simulink model "SF042A_HwAgSnsrls"  (R2013b)
settings: Solver=FixedStepDiscrete  SolverMode=SingleTasking  StartTime=0.0  StopTime=1  FixedStep=0.002  RelTol=1e-3
values from neighbouring files (symbols this model uses):
  ARCHGLBPRM_2MILLISEC_SEC_F32 = DataDict.Constant    [SF042A_HwAgSnsrls_DataDict.m]
  CORRDPINIONAGCON_CNT_U08 = DataDict.Constant    [SF042A_HwAgSnsrls_DataDict.m]
  FCENTROFFSCON_CNT_U08 = DataDict.Constant    [SF042A_HwAgSnsrls_DataDict.m]
  HwAgSnsrlsCorrdPinionAgHwConf = DataDict.Calibration    [SF042A_HwAgSnsrls_DataDict.m]
  HwAgSnsrlsFCentrHwConf = DataDict.Calibration    [SF042A_HwAgSnsrls_DataDict.m]
  HwAgSnsrlsSmotngCoeff = DataDict.Calibration    [SF042A_HwAgSnsrls_DataDict.m]
  HwAgSnsrlsSmotngStepThd = DataDict.Calibration    [SF042A_HwAgSnsrls_DataDict.m]
  HwAgSnsrlsStordPinionConf = DataDict.Calibration    [SF042A_HwAgSnsrls_DataDict.m]
  HwAgSnsrlsStordPinionConfThd = DataDict.Calibration    [SF042A_HwAgSnsrls_DataDict.m]
  HwAgSnsrlsVehDynDifThd = DataDict.Calibration    [SF042A_HwAgSnsrls_DataDict.m]
  HwAgSnsrlsVehDynHwConf = DataDict.Calibration    [SF042A_HwAgSnsrls_DataDict.m]
  HwAgSnsrlsVehDynMotVelThd = DataDict.Calibration    [SF042A_HwAgSnsrls_DataDict.m]
  HwAgSnsrlsVehDynPinionTqThd = DataDict.Calibration    [SF042A_HwAgSnsrls_DataDict.m]
  HwAgSnsrlsVehDynTmr1Thd = DataDict.Calibration    [SF042A_HwAgSnsrls_DataDict.m]
  HwAgSnsrlsVehDynTmr2Thd = DataDict.Calibration    [SF042A_HwAgSnsrls_DataDict.m]
  HwAgSnsrlsVehDynVehSpdThd = DataDict.Calibration    [SF042A_HwAgSnsrls_DataDict.m]
  HwAgSnsrlsVehDynYawRateThd = DataDict.Calibration    [SF042A_HwAgSnsrls_DataDict.m]
  HwAgSnsrlsWhlFrqThd = DataDict.Calibration    [SF042A_HwAgSnsrls_DataDict.m]
  HwAgSnsrlsWhlSpdHwAgCoeff1 = DataDict.Calibration    [SF042A_HwAgSnsrls_DataDict.m]
  HwAgSnsrlsWhlSpdHwAgCoeff2 = DataDict.Calibration    [SF042A_HwAgSnsrls_DataDict.m]
  HwAgSnsrlsWhlSpdHwAgThd = DataDict.Calibration    [SF042A_HwAgSnsrls_DataDict.m]
  HwAgSnsrlsWhlSpdHwConf = DataDict.Calibration    [SF042A_HwAgSnsrls_DataDict.m]
  HwAgSnsrlsWhlSpdRatThd = DataDict.Calibration    [SF042A_HwAgSnsrls_DataDict.m]
  HwAgSnsrlsWhlSpdTmrThd = DataDict.Calibration    [SF042A_HwAgSnsrls_DataDict.m]
  HwAgSnsrlsWhlSpdVehSpdThd = DataDict.Calibration    [SF042A_HwAgSnsrls_DataDict.m]
  LASTPOSNCON_CNT_U08 = DataDict.Constant    [SF042A_HwAgSnsrls_DataDict.m]
  MILLISECTO100MICROSEC_ULS_U32 = DataDict.Constant    [SF042A_HwAgSnsrls_DataDict.m]
  SysGlbPrmSysKineRat = DataDict.ImprtdCal    [SF042A_HwAgSnsrls_DataDict.m]
  SysGlbPrmSysTqRat = DataDict.ImprtdCal    [SF042A_HwAgSnsrls_DataDict.m]
  VEHDYNCON_CNT_U08 = DataDict.Constant    [SF042A_HwAgSnsrls_DataDict.m]
  WHLSPDCON_CNT_U08 = DataDict.Constant    [SF042A_HwAgSnsrls_DataDict.m]
undefined symbols (not defined in the file or in its folder): NtcNr1, SigQlfr1
libraries: NxtrAbslt x11, Fil x8, NxtrLim x4, simulink x3, NxtrNvM x1, FixdToFloat x1
(part 3 of 6)

== system SF042A_HwAgSnsrls/HwAgSnsrls/HwAgSnsrlsPer1/FCentr/If Action Subsystem ==
  RelHwAg : Inport  RequirementInfo={'linktype_rmi_doors' '00012961 (/E-STEER Core/SubSystem Specifications/Application Functions - EA4/SF042A Handwheel Angle Sensorless)' '#SF042A_69' 'true' 'REQ: SF042A_69' '' } %GIDa_4b6aed22_1d87_4b53_9189_d2644312f9f7
  Action Port : ActionPort  ActionType=then
  Constant1 : Constant  RequirementInfo="{'linktype_rmi_doors' '00012961 (/E-STEER Core/SubSystem Specifications/Application Functions - EA4/SF042A Handwheel Angle Sensorless)' '#SF042A_86' 'true' 'REQ:  SF042A_86' '' } %GIDa_2c467a3f_0d7c_4fdb_b837_6c4a5133068f"  Value=HwAgSnsrlsFCentrHwConf
  Constant2 : Constant  RequirementInfo={} %GIDa_675a5498_0baa_424c_b737_c1dad0f0e80d  Value=false  OutDataTypeStr=boolean
      settings: AttributesFormatString=%<OutDataTypeStr>
  CopyRight2 : Subsystem  Description=|  mask(Copyright Information){none=on}
      | Copyright info block.                                               
      |                                                                     
      | Place copyright information at the top of every subsystem in design.
      mask prompts: none "No parameters"
      mask help: Place copyright information at the top of every subsystem in design.
      mask Display:
      | NxtrConf = 'Nexteer Confidential';
      | 
      | sys = bdroot; %handle for the current model ("system")
      | first = get_param(sys,'Created');
      | if(isempty(first))
      |     first = datestr(now,'yyyy');
      | else
      |     first = first(end-3:end);  %year is last four digits
      | end
      | 
      | last = get_param(sys,'LastModifiedDate');
      | if isempty(last)
      |     last = datestr(now,'yyyy');
      | else
      |     last = last(end-3:end);
      | end
      | 
      | if strcmp(first,last)
      |     fprintf('%s -- Copyright %s Nexteer',NxtrConf,first)
      | else
      |     fprintf('%s -- %s%s- %s Nexteer',NxtrConf,char(169),first,last)
      | end
  Data Store Write : DataStoreWrite  RequirementInfo={} %GIDa_7ab1a69a_e36e_4ab1_a11e_792ec32a2170  DataStoreName=FCentrHwAgEna
  Data Store Write1 : DataStoreWrite  RequirementInfo={'linktype_rmi_doors' '00012961 (/E-STEER Core/SubSystem Specifications/Application Functions - EA4/SF042A Handwheel Angle Sensorless)' '#SF042A_69' 'true' 'REQ: SF042A_69' '' } %GIDa_34d06627_b66b_4ac4_8bdd_291c574c45f0  DataStoreName=FCentrHwAgOffs
  Data Store Write2 : DataStoreWrite  RequirementInfo="{'linktype_rmi_doors' '00012961 (/E-STEER Core/SubSystem Specifications/Application Functions - EA4/SF042A Handwheel Angle Sensorless)' '#SF042A_86' 'true' 'REQ:  SF042A_86' '' } %GIDa_6b896a4e_80c9_41a2_80ba_aa37785d56f0"  DataStoreName=FCentrHwConf
  wires:
  Constant1/1 -> Data Store Write2/1
  Constant2/1 -> Data Store Write/1
  RelHwAg/1 -> Data Store Write1/1

== system SF042A_HwAgSnsrls/HwAgSnsrls/HwAgSnsrlsPer1/RelHwAgCalcn/CopyRight2 ==

== system SF042A_HwAgSnsrls/HwAgSnsrls/HwAgSnsrlsPer1/RelHwAgCalcn/Set to 0 ==
  Action Port : ActionPort  ActionType=else
  Constant1 : Constant  RequirementInfo={} %GIDa_94a063b7_dc94_4966_ace2_3847eccd81e4  Value=0  OutDataTypeStr=single
      settings: AttributesFormatString=%<OutDataTypeStr>
  CopyRight2 : Subsystem  Description=|  mask(Copyright Information){none=on}
      | Copyright info block.                                               
      |                                                                     
      | Place copyright information at the top of every subsystem in design.
      mask prompts: none "No parameters"
      mask help: Place copyright information at the top of every subsystem in design.
      mask Display:
      | NxtrConf = 'Nexteer Confidential';
      | 
      | sys = bdroot; %handle for the current model ("system")
      | first = get_param(sys,'Created');
      | if(isempty(first))
      |     first = datestr(now,'yyyy');
      | else
      |     first = first(end-3:end);  %year is last four digits
      | end
      | 
      | last = get_param(sys,'LastModifiedDate');
      | if isempty(last)
      |     last = datestr(now,'yyyy');
      | else
      |     last = last(end-3:end);
      | end
      | 
      | if strcmp(first,last)
      |     fprintf('%s -- Copyright %s Nexteer',NxtrConf,first)
      | else
      |     fprintf('%s -- %s%s- %s Nexteer',NxtrConf,char(169),first,last)
      | end
  Out1 : Outport
  wires:
  Constant1/1 -> Out1/1

== system SF042A_HwAgSnsrls/HwAgSnsrls/HwAgSnsrlsPer1/RelHwAgCalcn/UseMotAg ==
  MotAgCumvAlgndCrf : Inport
  Action Port : ActionPort  ActionType=then
  CopyRight2 : Subsystem  Description=|  mask(Copyright Information){none=on}
      | Copyright info block.                                               
      |                                                                     
      | Place copyright information at the top of every subsystem in design.
      mask prompts: none "No parameters"
      mask help: Place copyright information at the top of every subsystem in design.
      mask Display:
      | NxtrConf = 'Nexteer Confidential';
      | 
      | sys = bdroot; %handle for the current model ("system")
      | first = get_param(sys,'Created');
      | if(isempty(first))
      |     first = datestr(now,'yyyy');
      | else
      |     first = first(end-3:end);  %year is last four digits
      | end
      | 
      | last = get_param(sys,'LastModifiedDate');
      | if isempty(last)
      |     last = datestr(now,'yyyy');
      | else
      |     last = last(end-3:end);
      | end
      | 
      | if strcmp(first,last)
      |     fprintf('%s -- Copyright %s Nexteer',NxtrConf,first)
      | else
      |     fprintf('%s -- %s%s- %s Nexteer',NxtrConf,char(169),first,last)
      | end
  Data Store Read2 : DataStoreRead  DataStoreName=MotAgOffsEna
  GetMotAgOffs : Subsystem  TreatAsAtomicUnit=on
  If : If  IfExpression=u1  ShowElse=off
  Out1 : Outport
  wires:
  MotAgCumvAlgndCrf/1 -> GetMotAgOffs/1(In1), Out1/1
  Data Store Read2/1 -> If/1
  If/1 -> GetMotAgOffs/Action

== system SF042A_HwAgSnsrls/HwAgSnsrls/HwAgSnsrlsPer1/Smoothing/CopyRight2 ==

== system SF042A_HwAgSnsrls/HwAgSnsrls/HwAgSnsrlsPer1/Smoothing/If Action Subsystem ==
  LrndHwAgDif : Inport
  Action Port : ActionPort  ActionType=then
  Add1 : Sum
  Constant1 : Constant  Value=true  OutDataTypeStr=boolean
  Constant3 : Constant  Value=HwAgSnsrlsSmotngCoeff
  CopyRight2 : Subsystem  Description=|  mask(Copyright Information){none=on}
      | Copyright info block.                                               
      |                                                                     
      | Place copyright information at the top of every subsystem in design.
      mask prompts: none "No parameters"
      mask help: Place copyright information at the top of every subsystem in design.
      mask Display:
      | NxtrConf = 'Nexteer Confidential';
      | 
      | sys = bdroot; %handle for the current model ("system")
      | first = get_param(sys,'Created');
      | if(isempty(first))
      |     first = datestr(now,'yyyy');
      | else
      |     first = first(end-3:end);  %year is last four digits
      | end
      | 
      | last = get_param(sys,'LastModifiedDate');
      | if isempty(last)
      |     last = datestr(now,'yyyy');
      | else
      |     last = last(end-3:end);
      | end
      | 
      | if strcmp(first,last)
      |     fprintf('%s -- Copyright %s Nexteer',NxtrConf,first)
      | else
      |     fprintf('%s -- %s%s- %s Nexteer',NxtrConf,char(169),first,last)
      | end
  Data Store Read2 : DataStoreRead  DataStoreName=PrevSmotngHwAg
  Data Store Write1 : DataStoreWrite  DataStoreName=PrevSmotngSt
  Product2 : Product
  Outp : Outport
  wires:
  Add1/1 -> Outp/1
  Product2/1 -> Add1/1
  Data Store Read2/1 -> Add1/2
  Constant3/1 -> Product2/2
  Constant1/1 -> Data Store Write1/1
  LrndHwAgDif/1 -> Product2/1

== system SF042A_HwAgSnsrls/HwAgSnsrls/HwAgSnsrlsPer1/Smoothing/If Action Subsystem1 ==
  LrndHwAg : Inport
  Action Port : ActionPort  ActionType=else
  Constant1 : Constant  Value=false  OutDataTypeStr=boolean
  CopyRight2 : Subsystem  Description=|  mask(Copyright Information){none=on}
      | Copyright info block.                                               
      |                                                                     
      | Place copyright information at the top of every subsystem in design.
      mask prompts: none "No parameters"
      mask help: Place copyright information at the top of every subsystem in design.
      mask Display:
      | NxtrConf = 'Nexteer Confidential';
      | 
      | sys = bdroot; %handle for the current model ("system")
      | first = get_param(sys,'Created');
      | if(isempty(first))
      |     first = datestr(now,'yyyy');
      | else
      |     first = first(end-3:end);  %year is last four digits
      | end
      | 
      | last = get_param(sys,'LastModifiedDate');
      | if isempty(last)
      |     last = datestr(now,'yyyy');
      | else
      |     last = last(end-3:end);
      | end
      | 
      | if strcmp(first,last)
      |     fprintf('%s -- Copyright %s Nexteer',NxtrConf,first)
      | else
      |     fprintf('%s -- %s%s- %s Nexteer',NxtrConf,char(169),first,last)
      | end
  Data Store Write1 : DataStoreWrite  DataStoreName=PrevSmotngSt
  Outp : Outport
  wires:
  LrndHwAg/1 -> Outp/1
  Constant1/1 -> Data Store Write1/1

== system SF042A_HwAgSnsrls/HwAgSnsrls/HwAgSnsrlsPer1/VehDynAutoCentr/CopyRight2 ==

== system SF042A_HwAgSnsrls/HwAgSnsrls/HwAgSnsrlsPer1/VehDynAutoCentr/LpFilOne ==
  FilOneEna : Inport
  RelHwAg : Inport  Port=2
  CopyRight2 : Subsystem  Description=|  mask(Copyright Information){none=on}
      | Copyright info block.                                               
      |                                                                     
      | Place copyright information at the top of every subsystem in design.
      mask prompts: none "No parameters"
      mask help: Place copyright information at the top of every subsystem in design.
      mask Display:
      | NxtrConf = 'Nexteer Confidential';
      | 
      | sys = bdroot; %handle for the current model ("system")
      | first = get_param(sys,'Created');
      | if(isempty(first))
      |     first = datestr(now,'yyyy');
      | else
      |     first = first(end-3:end);  %year is last four digits
      | end
      | 
      | last = get_param(sys,'LastModifiedDate');
      | if isempty(last)
      |     last = datestr(now,'yyyy');
      | else
      |     last = last(end-3:end);
      | end
      | 
      | if strcmp(first,last)
      |     fprintf('%s -- Copyright %s Nexteer',NxtrConf,first)
      | else
      |     fprintf('%s -- %s%s- %s Nexteer',NxtrConf,char(169),first,last)
      | end
  Data Store Write : DataStoreWrite  DataStoreName=PrevFildRelHwAg1
  If : If  RequirementInfo={'linktype_rmi_doors' '00012961 (/E-STEER Core/SubSystem Specifications/Application Functions - EA4/SF042A Handwheel Angle Sensorless)' '#SF042A_74' 'true' 'REQ: SF042A_74' '' } %GIDa_50dbe270_ec98_43d4_9cbb_cd5ecb0c86de  IfExpression=u1
  If Action Subsystem1 : Subsystem  RequirementInfo={'linktype_rmi_doors' '00012961 (/E-STEER Core/SubSystem Specifications/Application Functions - EA4/SF042A Handwheel Angle Sensorless)' '#SF042A_74' 'true' 'REQ: SF042A_74' '' } %GIDa_d396f57d_b9c8_4c45_ae6c_b596f7fbf48d  TreatAsAtomicUnit=on
  If Action Subsystem2 : Subsystem  RequirementInfo={'linktype_rmi_doors' '00012961 (/E-STEER Core/SubSystem Specifications/Application Functions - EA4/SF042A Handwheel Angle Sensorless)' '#SF042A_74' 'true' 'REQ: SF042A_74' '' } %GIDa_038cab70_eae8_4b9a_8597_cbcafc370d1a  TreatAsAtomicUnit=on
  Merge : Merge  RequirementInfo={'linktype_rmi_doors' '00012961 (/E-STEER Core/SubSystem Specifications/Application Functions - EA4/SF042A Handwheel Angle Sensorless)' '#SF042A_74' 'true' 'REQ: SF042A_74' '' } %GIDa_64de599a_2316_4355_972d_e88e49288b80
  FildRelHwAg1 : Outport
  wires:
  Merge/1 -> FildRelHwAg1/1, Data Store Write/1
  FilOneEna/1 -> If/1
  RelHwAg/1 -> If Action Subsystem2/1(RelHwAg)
  If Action Subsystem2/1(FildRelHwAg1) -> Merge/1
  If Action Subsystem1/1(FildRelHwAg1) -> Merge/2
  If/2 -> If Action Subsystem1/Action
  If/1 -> If Action Subsystem2/Action

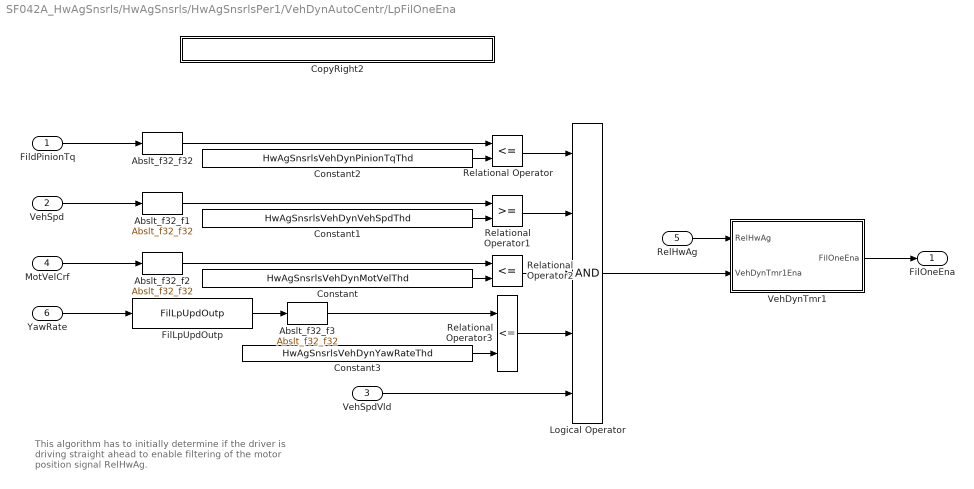
== system SF042A_HwAgSnsrls/HwAgSnsrls/HwAgSnsrlsPer1/VehDynAutoCentr/LpFilOneEna ==
  note: This algorithm has to initially determine if the driver is
      | driving straight ahead to enable filtering of the motor
      | position signal RelHwAg.
  FildPinionTq : Inport
  VehSpd : Inport  Port=2
  VehSpdVld : Inport  Port=3
  MotVelCrf : Inport  Port=4
  RelHwAg : Inport  Port=5
  YawRate : Inport  Port=6
  Abslt_f32_f1 : NxtrAbslt/Abslt_f32_f32  RequirementInfo={'linktype_rmi_doors' '00012961 (/E-STEER Core/SubSystem Specifications/Application Functions - EA4/SF042A Handwheel Angle Sensorless)' '#SF042A_73' 'true' 'REQ: SF042A_73' '' } %GIDa_47b4a5eb_74c9_48e6_977d_5f1b477ad6dd  SFunctionSpec=single y1 = Abslt_f32_f32(single u1)
      settings: AttributesFormatString=%<Name>
  Abslt_f32_f2 : NxtrAbslt/Abslt_f32_f32  RequirementInfo={'linktype_rmi_doors' '00012961 (/E-STEER Core/SubSystem Specifications/Application Functions - EA4/SF042A Handwheel Angle Sensorless)' '#SF042A_73' 'true' 'REQ: SF042A_73' '' } %GIDa_ea5515ef_69f8_4e78_8562_cc1ad73cd76b  SFunctionSpec=single y1 = Abslt_f32_f32(single u1)
      settings: AttributesFormatString=%<Name>
  Abslt_f32_f3 : NxtrAbslt/Abslt_f32_f32  RequirementInfo={'linktype_rmi_doors' '00012961 (/E-STEER Core/SubSystem Specifications/Application Functions - EA4/SF042A Handwheel Angle Sensorless)' '#SF042A_73' 'true' 'REQ: SF042A_73' '' } %GIDa_70050457_0f45_4f04_b196_a55d8517b918  SFunctionSpec=single y1 = Abslt_f32_f32(single u1)
      settings: AttributesFormatString=%<Name>
  Abslt_f32_f32 : NxtrAbslt/Abslt_f32_f32  RequirementInfo={'linktype_rmi_doors' '00012961 (/E-STEER Core/SubSystem Specifications/Application Functions - EA4/SF042A Handwheel Angle Sensorless)' '#SF042A_73' 'true' 'REQ: SF042A_73' '' } %GIDa_f624d835_a012_455e_a6e7_bf5bbda701df  SFunctionSpec=single y1 = Abslt_f32_f32(single u1)
      settings: AttributesFormatString=%<Name>
  Constant : Constant  RequirementInfo={'linktype_rmi_doors' '00012961 (/E-STEER Core/SubSystem Specifications/Application Functions - EA4/SF042A Handwheel Angle Sensorless)' '#SF042A_73' 'true' 'REQ: SF042A_73' '' } %GIDa_33de20e7_381d_4057_a25e_061ade792d0e  Value=HwAgSnsrlsVehDynMotVelThd
  Constant1 : Constant  RequirementInfo={'linktype_rmi_doors' '00012961 (/E-STEER Core/SubSystem Specifications/Application Functions - EA4/SF042A Handwheel Angle Sensorless)' '#SF042A_73' 'true' 'REQ: SF042A_73' '' } %GIDa_7455e53e_a0fa_4ad3_9554_8a19bfe16525  Value=HwAgSnsrlsVehDynVehSpdThd
  Constant2 : Constant  RequirementInfo={'linktype_rmi_doors' '00012961 (/E-STEER Core/SubSystem Specifications/Application Functions - EA4/SF042A Handwheel Angle Sensorless)' '#SF042A_73' 'true' 'REQ: SF042A_73' '' } %GIDa_60d6fec9_a19e_4266_9b3b_fb17078d585a  Value=HwAgSnsrlsVehDynPinionTqThd
  Constant3 : Constant  RequirementInfo={'linktype_rmi_doors' '00012961 (/E-STEER Core/SubSystem Specifications/Application Functions - EA4/SF042A Handwheel Angle Sensorless)' '#SF042A_73' 'true' 'REQ: SF042A_73' '' } %GIDa_08b4b183_3ae9_45ec_b5d2_fc4ee1e02481  Value=HwAgSnsrlsVehDynYawRateThd
  CopyRight2 : Subsystem  Description=|  mask(Copyright Information){none=on}
      | Copyright info block.                                               
      |                                                                     
      | Place copyright information at the top of every subsystem in design.
      mask prompts: none "No parameters"
      mask help: Place copyright information at the top of every subsystem in design.
      mask Display:
      | NxtrConf = 'Nexteer Confidential';
      | 
      | sys = bdroot; %handle for the current model ("system")
      | first = get_param(sys,'Created');
      | if(isempty(first))
      |     first = datestr(now,'yyyy');
      | else
      |     first = first(end-3:end);  %year is last four digits
      | end
      | 
      | last = get_param(sys,'LastModifiedDate');
      | if isempty(last)
      |     last = datestr(now,'yyyy');
      | else
      |     last = last(end-3:end);
      | end
      | 
      | if strcmp(first,last)
      |     fprintf('%s -- Copyright %s Nexteer',NxtrConf,first)
      | else
      |     fprintf('%s -- %s%s- %s Nexteer',NxtrConf,char(169),first,last)
      | end
  FilLpUpdOutp : Fil/FilLpUpdOutp  RequirementInfo={'linktype_rmi_doors' '00012961 (/E-STEER Core/SubSystem Specifications/Application Functions - EA4/SF042A Handwheel Angle Sensorless)' '#SF042A_73' 'true' 'REQ: SF042A_73' '' } %GIDa_2485b240_b275_4f39_b29a_c03896a8b7bb  StVar=YawRateFil
      settings: AttributesFormatString=StVar: %<StVar>
  Logical Operator : Logic  RequirementInfo={'linktype_rmi_doors' '00012961 (/E-STEER Core/SubSystem Specifications/Application Functions - EA4/SF042A Handwheel Angle Sensorless)' '#SF042A_73' 'true' 'REQ: SF042A_73' '' } %GIDa_490bb6e2_0097_4fb5_8883_f3aba4d42fa5  Inputs=5  AllPortsSameDT=off  OutDataTypeStr=boolean
  Relational Operator : RelationalOperator  RequirementInfo={'linktype_rmi_doors' '00012961 (/E-STEER Core/SubSystem Specifications/Application Functions - EA4/SF042A Handwheel Angle Sensorless)' '#SF042A_73' 'true' 'REQ: SF042A_73' '' } %GIDa_f6893bfc_cdd3_4f77_af64_1f833848b7e5  Operator=<=  OutDataTypeStr=boolean
  Relational Operator1 : RelationalOperator  RequirementInfo={'linktype_rmi_doors' '00012961 (/E-STEER Core/SubSystem Specifications/Application Functions - EA4/SF042A Handwheel Angle Sensorless)' '#SF042A_73' 'true' 'REQ: SF042A_73' '' } %GIDa_8a3715e6_0a30_4e30_a0ce_0eaccb932bbf  OutDataTypeStr=boolean
  Relational Operator2 : RelationalOperator  RequirementInfo={'linktype_rmi_doors' '00012961 (/E-STEER Core/SubSystem Specifications/Application Functions - EA4/SF042A Handwheel Angle Sensorless)' '#SF042A_73' 'true' 'REQ: SF042A_73' '' } %GIDa_3da8d1a4_697d_4093_b262_91d6ea858a11  Operator=<=  OutDataTypeStr=boolean
  Relational Operator3 : RelationalOperator  RequirementInfo={'linktype_rmi_doors' '00012961 (/E-STEER Core/SubSystem Specifications/Application Functions - EA4/SF042A Handwheel Angle Sensorless)' '#SF042A_73' 'true' 'REQ: SF042A_73' '' } %GIDa_40a0aebf_3696_464f_8498_1d8daec05661  Operator=<=  OutDataTypeStr=boolean
  VehDynTmr1 : Subsystem  RequirementInfo={'linktype_rmi_doors' '00012961 (/E-STEER Core/SubSystem Specifications/Application Functions - EA4/SF042A Handwheel Angle Sensorless)' '#SF042A_73' 'true' 'REQ: SF042A_73' '' } %GIDa_9b420d72_230e_42ee_a755_3d84b38ed0e9
  FilOneEna : Outport
  wires:
  Abslt_f32_f3/1 -> Relational Operator3/1
  VehSpdVld/1 -> Logical Operator/5
  Constant3/1 -> Relational Operator3/2
  FilLpUpdOutp/1 -> Abslt_f32_f3/1
  YawRate/1 -> FilLpUpdOutp/1
  Logical Operator/1 -> VehDynTmr1/2(VehDynTmr1Ena)
  VehDynTmr1/1(FilOneEna) -> FilOneEna/1
  RelHwAg/1 -> VehDynTmr1/1(RelHwAg)
  Relational Operator2/1 -> Logical Operator/3
  Relational Operator1/1 -> Logical Operator/2
  Relational Operator/1 -> Logical Operator/1
  Relational Operator3/1 -> Logical Operator/4
  Abslt_f32_f2/1 -> Relational Operator2/1
  Constant/1 -> Relational Operator2/2
  Abslt_f32_f1/1 -> Relational Operator1/1
  Constant1/1 -> Relational Operator1/2
  VehSpd/1 -> Abslt_f32_f1/1
  Abslt_f32_f32/1 -> Relational Operator/1
  Constant2/1 -> Relational Operator/2
  MotVelCrf/1 -> Abslt_f32_f2/1
  FildPinionTq/1 -> Abslt_f32_f32/1

== system SF042A_HwAgSnsrls/HwAgSnsrls/HwAgSnsrlsPer1/VehDynAutoCentr/LpFilTwo ==
  note: The output, VehDynHwAg is removed.
      | The display, dHwAgSnsrlsVehDynHwAg is removed.
      | The PIM, PrevFildRelHwAg2 is removed.
  FilTwoEna : Inport
  RelHwAg : Inport  Port=2
  CopyRight2 : Subsystem  Description=|  mask(Copyright Information){none=on}
      | Copyright info block.                                               
      |                                                                     
      | Place copyright information at the top of every subsystem in design.
      mask prompts: none "No parameters"
      mask help: Place copyright information at the top of every subsystem in design.
      mask Display:
      | NxtrConf = 'Nexteer Confidential';
      | 
      | sys = bdroot; %handle for the current model ("system")
      | first = get_param(sys,'Created');
      | if(isempty(first))
      |     first = datestr(now,'yyyy');
      | else
      |     first = first(end-3:end);  %year is last four digits
      | end
      | 
      | last = get_param(sys,'LastModifiedDate');
      | if isempty(last)
      |     last = datestr(now,'yyyy');
      | else
      |     last = last(end-3:end);
      | end
      | 
      | if strcmp(first,last)
      |     fprintf('%s -- Copyright %s Nexteer',NxtrConf,first)
      | else
      |     fprintf('%s -- %s%s- %s Nexteer',NxtrConf,char(169),first,last)
      | end
  Data Store Write1 : DataStoreWrite  DataStoreName=dHwAgSnsrlsVehDynHwConf
  If Action Subsystem3 : Subsystem  RequirementInfo={'linktype_rmi_doors' '00012961 (/E-STEER Core/SubSystem Specifications/Application Functions - EA4/SF042A Handwheel Angle Sensorless)' '#SF042A_76' 'true' 'REQ: SF042A_76' '' } %GIDa_7c18b11c_08c4_4ee8_9dc5_2a8c731949f7  TreatAsAtomicUnit=on
  If Action Subsystem4 : Subsystem  RequirementInfo={'linktype_rmi_doors' '00012961 (/E-STEER Core/SubSystem Specifications/Application Functions - EA4/SF042A Handwheel Angle Sensorless)' '#SF042A_77' 'true' 'REQ: SF042A_77' '' } %GIDa_7dd1b9c8_568d_422e_9620_51905b8cb554  TreatAsAtomicUnit=on
  If1 : If  RequirementInfo={'linktype_rmi_doors' '00012961 (/E-STEER Core/SubSystem Specifications/Application Functions - EA4/SF042A Handwheel Angle Sensorless)' '#SF042A_76' 'true' 'REQ: SF042A_76' '' ; 'linktype_rmi_doors' '00012961 (/E-STEER Core/SubSystem Specifications/Application Functions - EA4/SF042A Handwheel Angle Sensorless)' '#SF042A_77' 'true' 'REQ: SF042A_77' '' } %GIDa_16361238_c0a5_470c_9b94_2028cab79145  IfExpression=u1
  Merge2 : Merge  RequirementInfo={'linktype_rmi_doors' '00012961 (/E-STEER Core/SubSystem Specifications/Application Functions - EA4/SF042A Handwheel Angle Sensorless)' '#SF042A_76' 'true' 'REQ: SF042A_76' '' ; 'linktype_rmi_doors' '00012961 (/E-STEER Core/SubSystem Specifications/Application Functions - EA4/SF042A Handwheel Angle Sensorless)' '#SF042A_77' 'true' 'REQ: SF042A_77' '' } %GIDa_e93193e5_4d94_47be_88ff_d96e66fc9642
  VehDynHwConf : Outport
  wires:
  Merge2/1 -> VehDynHwConf/1, Data Store Write1/1
  If Action Subsystem4/1(VehDynHwConf) -> Merge2/1
  If Action Subsystem3/1(VehDynHwConf) -> Merge2/2
  FilTwoEna/1 -> If1/1
  RelHwAg/1 -> If Action Subsystem4/1(RelHwAg)
  If1/1 -> If Action Subsystem4/Action
  If1/2 -> If Action Subsystem3/Action

== system SF042A_HwAgSnsrls/HwAgSnsrls/HwAgSnsrlsPer1/VehDynAutoCentr/LpFilTwoEna ==
  FildRelHwAg1 : Inport
  RelHwAg : Inport  Port=2
  FilOneEna : Inport  Port=3
  Abslt_f32_f3 : NxtrAbslt/Abslt_f32_f32  RequirementInfo={'linktype_rmi_doors' '00012961 (/E-STEER Core/SubSystem Specifications/Application Functions - EA4/SF042A Handwheel Angle Sensorless)' '#SF042A_75' 'true' 'REQ: SF042A_75' '' } %GIDa_6aeccc63_8826_4a9a_b358_b34695279e3a  SFunctionSpec=single y1 = Abslt_f32_f32(single u1)
      settings: AttributesFormatString=%<Name>
  Add : Sum  RequirementInfo={'linktype_rmi_doors' '00012961 (/E-STEER Core/SubSystem Specifications/Application Functions - EA4/SF042A Handwheel Angle Sensorless)' '#SF042A_75' 'true' 'REQ: SF042A_75' '' } %GIDa_bed5965e_f792_4fe9_be9c_a249f6adb978  Inputs=-+
  Constant5 : Constant  RequirementInfo={'linktype_rmi_doors' '00012961 (/E-STEER Core/SubSystem Specifications/Application Functions - EA4/SF042A Handwheel Angle Sensorless)' '#SF042A_75' 'true' 'REQ: SF042A_75' '' } %GIDa_4312dcf7_970c_416a_83c8_6d334342d5f4  Value=HwAgSnsrlsVehDynDifThd
  CopyRight2 : Subsystem  Description=|  mask(Copyright Information){none=on}
      | Copyright info block.                                               
      |                                                                     
      | Place copyright information at the top of every subsystem in design.
      mask prompts: none "No parameters"
      mask help: Place copyright information at the top of every subsystem in design.
      mask Display:
      | NxtrConf = 'Nexteer Confidential';
      | 
      | sys = bdroot; %handle for the current model ("system")
      | first = get_param(sys,'Created');
      | if(isempty(first))
      |     first = datestr(now,'yyyy');
      | else
      |     first = first(end-3:end);  %year is last four digits
      | end
      | 
      | last = get_param(sys,'LastModifiedDate');
      | if isempty(last)
      |     last = datestr(now,'yyyy');
      | else
      |     last = last(end-3:end);
      | end
      | 
      | if strcmp(first,last)
      |     fprintf('%s -- Copyright %s Nexteer',NxtrConf,first)
      | else
      |     fprintf('%s -- %s%s- %s Nexteer',NxtrConf,char(169),first,last)
      | end
  Logical Operator1 : Logic  RequirementInfo={'linktype_rmi_doors' '00012961 (/E-STEER Core/SubSystem Specifications/Application Functions - EA4/SF042A Handwheel Angle Sensorless)' '#SF042A_75' 'true' 'REQ: SF042A_75' '' } %GIDa_69a84b1a_4e75_466e_ae3a_2b9fc6914824  AllPortsSameDT=off  OutDataTypeStr=boolean
  Relational Operator3 : RelationalOperator  RequirementInfo={'linktype_rmi_doors' '00012961 (/E-STEER Core/SubSystem Specifications/Application Functions - EA4/SF042A Handwheel Angle Sensorless)' '#SF042A_75' 'true' 'REQ: SF042A_75' '' } %GIDa_439f62f5_372d_47fa_800c_5b377eb6c5df  Operator=<=  OutDataTypeStr=boolean
  VehDynTmr2 : Subsystem  RequirementInfo={'linktype_rmi_doors' '00012961 (/E-STEER Core/SubSystem Specifications/Application Functions - EA4/SF042A Handwheel Angle Sensorless)' '#SF042A_75' 'true' 'REQ: SF042A_75' '' } %GIDa_bc352537_dcd2_4910_87c3_9f7bc64451ab
  FilTwoEna : Outport
  wires:
  FildRelHwAg1/1 -> Add/1, [FildRelHwAg1]
  VehDynTmr2/1(FilTwoEna) -> FilTwoEna/1
  [FildRelHwAg1] -> VehDynTmr2/1(FildRelHwAg1)
  Logical Operator1/1 -> VehDynTmr2/2(VehDynTmr2Ena)
  FilOneEna/1 -> Logical Operator1/2
  Relational Operator3/1 -> Logical Operator1/1
  Constant5/1 -> Relational Operator3/2
  Abslt_f32_f3/1 -> Relational Operator3/1
  Add/1 -> Abslt_f32_f3/1
  RelHwAg/1 -> Add/2

== system SF042A_HwAgSnsrls/HwAgSnsrls/HwAgSnsrlsPer1/VehDynAutoCentr/PinionTqCalc ==
  HwTq : Inport
  MotTqCmdCrf : Inport  Port=2
  Add : Sum  RequirementInfo={'linktype_rmi_doors' '00012961 (/E-STEER Core/SubSystem Specifications/Application Functions - EA4/SF042A Handwheel Angle Sensorless)' '#SF042A_67' 'true' 'REQ: SF042A_67' '' } %GIDa_29639fb6_7c22_449f_aaa9_e717a68ba06e
  Constant : Constant  RequirementInfo={'linktype_rmi_doors' '00012961 (/E-STEER Core/SubSystem Specifications/Application Functions - EA4/SF042A Handwheel Angle Sensorless)' '#SF042A_67' 'true' 'REQ: SF042A_67' '' } %GIDa_ce2a4e4e_2b87_4ac6_9ab1_d2b13d4c852e  Value=SysGlbPrmSysTqRat
  CopyRight2 : Subsystem  Description=|  mask(Copyright Information){none=on}
      | Copyright info block.                                               
      |                                                                     
      | Place copyright information at the top of every subsystem in design.
      mask prompts: none "No parameters"
      mask help: Place copyright information at the top of every subsystem in design.
      mask Display:
      | NxtrConf = 'Nexteer Confidential';
      | 
      | sys = bdroot; %handle for the current model ("system")
      | first = get_param(sys,'Created');
      | if(isempty(first))
      |     first = datestr(now,'yyyy');
      | else
      |     first = first(end-3:end);  %year is last four digits
      | end
      | 
      | last = get_param(sys,'LastModifiedDate');
      | if isempty(last)
      |     last = datestr(now,'yyyy');
      | else
      |     last = last(end-3:end);
      | end
      | 
      | if strcmp(first,last)
      |     fprintf('%s -- Copyright %s Nexteer',NxtrConf,first)
      | else
      |     fprintf('%s -- %s%s- %s Nexteer',NxtrConf,char(169),first,last)
      | end
  FilLpUpdOutp : Fil/FilLpUpdOutp  RequirementInfo={'linktype_rmi_doors' '00012961 (/E-STEER Core/SubSystem Specifications/Application Functions - EA4/SF042A Handwheel Angle Sensorless)' '#SF042A_67' 'true' 'REQ: SF042A_67' '' } %GIDa_71b12ad7_8a05_45a2_a00d_d65e9feee573  StVar=PinionTqFil
      settings: AttributesFormatString=StVar: %<StVar>
  Product : Product  RequirementInfo={'linktype_rmi_doors' '00012961 (/E-STEER Core/SubSystem Specifications/Application Functions - EA4/SF042A Handwheel Angle Sensorless)' '#SF042A_67' 'true' 'REQ: SF042A_67' '' } %GIDa_12316cbc_e5f8_4b38_99f2_690332d89a1e
  FildPinionTq : Outport
  wires:
  Constant/1 -> Product/2
  FilLpUpdOutp/1 -> FildPinionTq/1
  Add/1 -> FilLpUpdOutp/1
  HwTq/1 -> Add/1
  Product/1 -> Add/2
  MotTqCmdCrf/1 -> Product/1

== system SF042A_HwAgSnsrls/HwAgSnsrls/HwAgSnsrlsPer1/WhlSpdAutoCentr/CopyRight2 ==

== system SF042A_HwAgSnsrls/HwAgSnsrls/HwAgSnsrlsPer1/WhlSpdAutoCentr/WhlFrqNotVld ==
  note: The output, WhlSpdHwAg, is removed.
  Action Port : ActionPort  ActionType=else
  Constant1 : Constant  Value=0  OutDataTypeStr=single
      settings: AttributesFormatString=%<OutDataTypeStr>
  CopyRight2 : Subsystem  Description=|  mask(Copyright Information){none=on}
      | Copyright info block.                                               
      |                                                                     
      | Place copyright information at the top of every subsystem in design.
      mask prompts: none "No parameters"
      mask help: Place copyright information at the top of every subsystem in design.
      mask Display:
      | NxtrConf = 'Nexteer Confidential';
      | 
      | sys = bdroot; %handle for the current model ("system")
      | first = get_param(sys,'Created');
      | if(isempty(first))
      |     first = datestr(now,'yyyy');
      | else
      |     first = first(end-3:end);  %year is last four digits
      | end
      | 
      | last = get_param(sys,'LastModifiedDate');
      | if isempty(last)
      |     last = datestr(now,'yyyy');
      | else
      |     last = last(end-3:end);
      | end
      | 
      | if strcmp(first,last)
      |     fprintf('%s -- Copyright %s Nexteer',NxtrConf,first)
      | else
      |     fprintf('%s -- %s%s- %s Nexteer',NxtrConf,char(169),first,last)
      | end
  WhlSpdHwConf : Outport
  wires:
  Constant1/1 -> WhlSpdHwConf/1

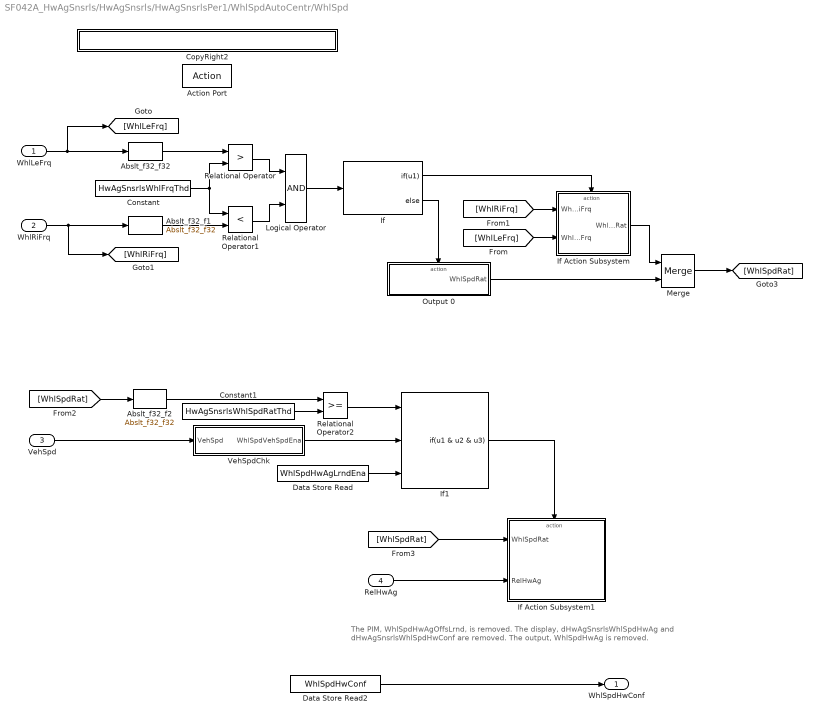
== system SF042A_HwAgSnsrls/HwAgSnsrls/HwAgSnsrlsPer1/WhlSpdAutoCentr/WhlSpd ==
  note: The PIM, WhlSpdHwAgOffsLrnd, is removed.
      | The display, dHwAgSnsrlsWhlSpdHwAg and dHwAgSnsrlsWhlSpdHwConf are removed.
      | The output, WhlSpdHwAg is removed.
  WhlLeFrq : Inport
  WhlRiFrq : Inport  Port=2
  VehSpd : Inport  Port=3
  RelHwAg : Inport  Port=4
  Action Port : ActionPort  ActionType=then
  Abslt_f32_f1 : NxtrAbslt/Abslt_f32_f32  RequirementInfo={'linktype_rmi_doors' '00012961 (/E-STEER Core/SubSystem Specifications/Application Functions - EA4/SF042A Handwheel Angle Sensorless)' '#SF042A_65' 'true' 'REQ: SF042A_65' '' } %GIDa_d4aa8001_83fa_4c6f_9809_89a43d8aca27  SFunctionSpec=single y1 = Abslt_f32_f32(single u1)
      settings: AttributesFormatString=%<Name>
  Abslt_f32_f2 : NxtrAbslt/Abslt_f32_f32  RequirementInfo={'linktype_rmi_doors' '00012961 (/E-STEER Core/SubSystem Specifications/Application Functions - EA4/SF042A Handwheel Angle Sensorless)' '#SF042A_70' 'true' 'REQ: SF042A_70' '' } %GIDa_5792167f_9657_46b9_be46_677adbbbb6ab  SFunctionSpec=single y1 = Abslt_f32_f32(single u1)
      settings: AttributesFormatString=%<Name>
  Abslt_f32_f32 : NxtrAbslt/Abslt_f32_f32  RequirementInfo={'linktype_rmi_doors' '00012961 (/E-STEER Core/SubSystem Specifications/Application Functions - EA4/SF042A Handwheel Angle Sensorless)' '#SF042A_65' 'true' 'REQ: SF042A_65' '' } %GIDa_e64233e3_8490_43e3_9bb9_b1c1de4864fc  SFunctionSpec=single y1 = Abslt_f32_f32(single u1)
      settings: AttributesFormatString=%<Name>
  Constant : Constant  RequirementInfo={'linktype_rmi_doors' '00012961 (/E-STEER Core/SubSystem Specifications/Application Functions - EA4/SF042A Handwheel Angle Sensorless)' '#SF042A_65' 'true' 'REQ: SF042A_65' '' } %GIDa_7d4b8ce5_25b7_4474_9e59_28dcb7bee1cc  Value=HwAgSnsrlsWhlFrqThd
  Constant1 : Constant  RequirementInfo={'linktype_rmi_doors' '00012961 (/E-STEER Core/SubSystem Specifications/Application Functions - EA4/SF042A Handwheel Angle Sensorless)' '#SF042A_70' 'true' 'REQ: SF042A_70' '' } %GIDa_189f23fb_e9e8_4ae2_b5ff_0cfeb2022c31  Value=HwAgSnsrlsWhlSpdRatThd
  CopyRight2 : Subsystem  Description=|  mask(Copyright Information){none=on}
      | Copyright info block.                                               
      |                                                                     
      | Place copyright information at the top of every subsystem in design.
      mask prompts: none "No parameters"
      mask help: Place copyright information at the top of every subsystem in design.
      mask Display:
      | NxtrConf = 'Nexteer Confidential';
      | 
      | sys = bdroot; %handle for the current model ("system")
      | first = get_param(sys,'Created');
      | if(isempty(first))
      |     first = datestr(now,'yyyy');
      | else
      |     first = first(end-3:end);  %year is last four digits
      | end
      | 
      | last = get_param(sys,'LastModifiedDate');
      | if isempty(last)
      |     last = datestr(now,'yyyy');
      | else
      |     last = last(end-3:end);
      | end
      | 
      | if strcmp(first,last)
      |     fprintf('%s -- Copyright %s Nexteer',NxtrConf,first)
      | else
      |     fprintf('%s -- %s%s- %s Nexteer',NxtrConf,char(169),first,last)
      | end
  Data Store Read : DataStoreRead  RequirementInfo={'linktype_rmi_doors' '00012961 (/E-STEER Core/SubSystem Specifications/Application Functions - EA4/SF042A Handwheel Angle Sensorless)' '#SF042A_70' 'true' 'REQ: SF042A_70' '' } %GIDa_68a56ab5_0222_4cbb_a5e5_dfbe2b8a8f10  DataStoreName=WhlSpdHwAgLrndEna
  Data Store Read2 : DataStoreRead  DataStoreName=WhlSpdHwConf
  If : If  RequirementInfo={'linktype_rmi_doors' '00012961 (/E-STEER Core/SubSystem Specifications/Application Functions - EA4/SF042A Handwheel Angle Sensorless)' '#SF042A_65' 'true' 'REQ: SF042A_65' '' } %GIDa_2e876f49_124f_4183_885a_3dea6b3dad2f  IfExpression=u1
  If Action Subsystem : Subsystem  RequirementInfo={'linktype_rmi_doors' '00012961 (/E-STEER Core/SubSystem Specifications/Application Functions - EA4/SF042A Handwheel Angle Sensorless)' '#SF042A_65' 'true' 'REQ: SF042A_65' '' } %GIDa_899061f6_d096_4124_b49c_fcc09747206b  TreatAsAtomicUnit=on
  If Action Subsystem1 : Subsystem  RequirementInfo={'linktype_rmi_doors' '00012961 (/E-STEER Core/SubSystem Specifications/Application Functions - EA4/SF042A Handwheel Angle Sensorless)' '#SF042A_70' 'true' 'REQ: SF042A_70' '' } %GIDa_1019010c_5c1d_4394_9265_225bf7011aeb  TreatAsAtomicUnit=on
  If1 : If  RequirementInfo={'linktype_rmi_doors' '00012961 (/E-STEER Core/SubSystem Specifications/Application Functions - EA4/SF042A Handwheel Angle Sensorless)' '#SF042A_70' 'true' 'REQ: SF042A_70' '' } %GIDa_72af7a9f_00c7_4a9b_9e53_e7e02b2d58d3  NumInputs=3  IfExpression=u1 & u2 & u3  ShowElse=off
  Logical Operator : Logic  RequirementInfo={'linktype_rmi_doors' '00012961 (/E-STEER Core/SubSystem Specifications/Application Functions - EA4/SF042A Handwheel Angle Sensorless)' '#SF042A_65' 'true' 'REQ: SF042A_65' '' } %GIDa_6d13c416_37b1_4a1b_94e2_89b1756b671c  AllPortsSameDT=off  OutDataTypeStr=boolean
  Merge : Merge  RequirementInfo={'linktype_rmi_doors' '00012961 (/E-STEER Core/SubSystem Specifications/Application Functions - EA4/SF042A Handwheel Angle Sensorless)' '#SF042A_65' 'true' 'REQ: SF042A_65' '' } %GIDa_a970084c_f16c_449d_a4e4_d262d14d37c3
  Output 0 : Subsystem  RequirementInfo={'linktype_rmi_doors' '00012961 (/E-STEER Core/SubSystem Specifications/Application Functions - EA4/SF042A Handwheel Angle Sensorless)' '#SF042A_65' 'true' 'REQ: SF042A_65' '' } %GIDa_cec3c8a0_c03e_495a_8c57_f553e2171421  TreatAsAtomicUnit=on
  Relational Operator : RelationalOperator  RequirementInfo={'linktype_rmi_doors' '00012961 (/E-STEER Core/SubSystem Specifications/Application Functions - EA4/SF042A Handwheel Angle Sensorless)' '#SF042A_65' 'true' 'REQ: SF042A_65' '' } %GIDa_489c5c79_b489_4020_9f52_07b314a04812  Operator=>  OutDataTypeStr=boolean
  Relational Operator1 : RelationalOperator  RequirementInfo={'linktype_rmi_doors' '00012961 (/E-STEER Core/SubSystem Specifications/Application Functions - EA4/SF042A Handwheel Angle Sensorless)' '#SF042A_65' 'true' 'REQ: SF042A_65' '' } %GIDa_963dfc29_7ca3_4c5f_874f_6035a82b480f  Operator=<  OutDataTypeStr=boolean
  Relational Operator2 : RelationalOperator  RequirementInfo={'linktype_rmi_doors' '00012961 (/E-STEER Core/SubSystem Specifications/Application Functions - EA4/SF042A Handwheel Angle Sensorless)' '#SF042A_70' 'true' 'REQ: SF042A_70' '' } %GIDa_74815e4d_93dc_48c6_9140_62f50d698ab8  OutDataTypeStr=boolean
  VehSpdChk : Subsystem  RequirementInfo={'linktype_rmi_doors' '00012961 (/E-STEER Core/SubSystem Specifications/Application Functions - EA4/SF042A Handwheel Angle Sensorless)' '#SF042A_70' 'true' 'REQ: SF042A_70' '' } %GIDa_d063fdf7_7de5_474b_886a_3704cb97dafd
  WhlSpdHwConf : Outport
  wires:
  Data Store Read/1 -> If1/3
  RelHwAg/1 -> If Action Subsystem1/2(RelHwAg)
  Data Store Read2/1 -> WhlSpdHwConf/1
  WhlLeFrq/1 -> Abslt_f32_f32/1, [WhlLeFrq]
  Abslt_f32_f32/1 -> Relational Operator/1
  Abslt_f32_f1/1 -> Relational Operator1/2
  Constant/1 -> Relational Operator/2, Relational Operator1/1
  Relational Operator/1 -> Logical Operator/1
  Relational Operator1/1 -> Logical Operator/2
  Logical Operator/1 -> If/1
  If/1 -> If Action Subsystem/Action
  If/2 -> Output 0/Action
  WhlRiFrq/1 -> [WhlRiFrq], Abslt_f32_f1/1
  [WhlRiFrq] -> If Action Subsystem/1(WhlRiFrq)
  [WhlLeFrq] -> If Action Subsystem/2(WhlLeFrq)
  Merge/1 -> [WhlSpdRat]
  Output 0/1(WhlSpdRat) -> Merge/2
  If Action Subsystem/1(WhlSpdRat) -> Merge/1
  [WhlSpdRat] -> Abslt_f32_f2/1
  Abslt_f32_f2/1 -> Relational Operator2/1
  Constant1/1 -> Relational Operator2/2
  Relational Operator2/1 -> If1/1
  If1/1 -> If Action Subsystem1/Action
  [WhlSpdRat] -> If Action Subsystem1/1(WhlSpdRat)
  VehSpd/1 -> VehSpdChk/1(VehSpd)
  VehSpdChk/1(WhlSpdVehSpdEna) -> If1/2

== system SF042A_HwAgSnsrls/HwAgSnsrls/HwAgSnsrlsPer1/Arbitrator/MaxHwConf/CopyRight2 ==

== system SF042A_HwAgSnsrls/HwAgSnsrls/HwAgSnsrlsPer1/Arbitrator/MaxHwConf/If Action Subsystem ==
  FCentrHwConf : Inport
  Action Port : ActionPort  ActionType=then
  Constant1 : Constant  Value=FCENTROFFSCON_CNT_U08
  CopyRight2 : Subsystem  Description=|  mask(Copyright Information){none=on}
      | Copyright info block.                                               
      |                                                                     
      | Place copyright information at the top of every subsystem in design.
      mask prompts: none "No parameters"
      mask help: Place copyright information at the top of every subsystem in design.
      mask Display:
      | NxtrConf = 'Nexteer Confidential';
      | 
      | sys = bdroot; %handle for the current model ("system")
      | first = get_param(sys,'Created');
      | if(isempty(first))
      |     first = datestr(now,'yyyy');
      | else
      |     first = first(end-3:end);  %year is last four digits
      | end
      | 
      | last = get_param(sys,'LastModifiedDate');
      | if isempty(last)
      |     last = datestr(now,'yyyy');
      | else
      |     last = last(end-3:end);
      | end
      | 
      | if strcmp(first,last)
      |     fprintf('%s -- Copyright %s Nexteer',NxtrConf,first)
      | else
      |     fprintf('%s -- %s%s- %s Nexteer',NxtrConf,char(169),first,last)
      | end
  MaxHwConf1 : Outport
  SelnCaseSt1 : Outport  Port=2
  wires:
  FCentrHwConf/1 -> MaxHwConf1/1
  Constant1/1 -> SelnCaseSt1/1

== system SF042A_HwAgSnsrls/HwAgSnsrls/HwAgSnsrlsPer1/Arbitrator/MaxHwConf/If Action Subsystem1 ==
  VehDynHwConf : Inport
  Action Port : ActionPort  ActionType=else
  Constant2 : Constant  Value=VEHDYNCON_CNT_U08
  CopyRight2 : Subsystem  Description=|  mask(Copyright Information){none=on}
      | Copyright info block.                                               
      |                                                                     
      | Place copyright information at the top of every subsystem in design.
      mask prompts: none "No parameters"
      mask help: Place copyright information at the top of every subsystem in design.
      mask Display:
      | NxtrConf = 'Nexteer Confidential';
      | 
      | sys = bdroot; %handle for the current model ("system")
      | first = get_param(sys,'Created');
      | if(isempty(first))
      |     first = datestr(now,'yyyy');
      | else
      |     first = first(end-3:end);  %year is last four digits
      | end
      | 
      | last = get_param(sys,'LastModifiedDate');
      | if isempty(last)
      |     last = datestr(now,'yyyy');
      | else
      |     last = last(end-3:end);
      | end
      | 
      | if strcmp(first,last)
      |     fprintf('%s -- Copyright %s Nexteer',NxtrConf,first)
      | else
      |     fprintf('%s -- %s%s- %s Nexteer',NxtrConf,char(169),first,last)
      | end
  MaxHwConf1 : Outport
  SelnCaseSt1 : Outport  Port=2
  wires:
  VehDynHwConf/1 -> MaxHwConf1/1
  Constant2/1 -> SelnCaseSt1/1

== system SF042A_HwAgSnsrls/HwAgSnsrls/HwAgSnsrlsPer1/Arbitrator/MaxHwConf/If Action Subsystem2 ==
  MaxHwConf1 : Inport
  SelnCaseSt1 : Inport  Port=2
  Action Port : ActionPort  ActionType=then
  CopyRight2 : Subsystem  Description=|  mask(Copyright Information){none=on}
      | Copyright info block.                                               
      |                                                                     
      | Place copyright information at the top of every subsystem in design.
      mask prompts: none "No parameters"
      mask help: Place copyright information at the top of every subsystem in design.
      mask Display:
      | NxtrConf = 'Nexteer Confidential';
      | 
      | sys = bdroot; %handle for the current model ("system")
      | first = get_param(sys,'Created');
      | if(isempty(first))
      |     first = datestr(now,'yyyy');
      | else
      |     first = first(end-3:end);  %year is last four digits
      | end
      | 
      | last = get_param(sys,'LastModifiedDate');
      | if isempty(last)
      |     last = datestr(now,'yyyy');
      | else
      |     last = last(end-3:end);
      | end
      | 
      | if strcmp(first,last)
      |     fprintf('%s -- Copyright %s Nexteer',NxtrConf,first)
      | else
      |     fprintf('%s -- %s%s- %s Nexteer',NxtrConf,char(169),first,last)
      | end
  MaxHwConf3 : Outport
  SelnCaseSt3 : Outport  Port=2
  wires:
  MaxHwConf1/1 -> MaxHwConf3/1
  SelnCaseSt1/1 -> SelnCaseSt3/1

== system SF042A_HwAgSnsrls/HwAgSnsrls/HwAgSnsrlsPer1/Arbitrator/MaxHwConf/If Action Subsystem3 ==
  MaxHwConf2 : Inport
  SelnCaseSt2 : Inport  Port=2
  Action Port : ActionPort  ActionType=else
  CopyRight2 : Subsystem  Description=|  mask(Copyright Information){none=on}
      | Copyright info block.                                               
      |                                                                     
      | Place copyright information at the top of every subsystem in design.
      mask prompts: none "No parameters"
      mask help: Place copyright information at the top of every subsystem in design.
      mask Display:
      | NxtrConf = 'Nexteer Confidential';
      | 
      | sys = bdroot; %handle for the current model ("system")
      | first = get_param(sys,'Created');
      | if(isempty(first))
      |     first = datestr(now,'yyyy');
      | else
      |     first = first(end-3:end);  %year is last four digits
      | end
      | 
      | last = get_param(sys,'LastModifiedDate');
      | if isempty(last)
      |     last = datestr(now,'yyyy');
      | else
      |     last = last(end-3:end);
      | end
      | 
      | if strcmp(first,last)
      |     fprintf('%s -- Copyright %s Nexteer',NxtrConf,first)
      | else
      |     fprintf('%s -- %s%s- %s Nexteer',NxtrConf,char(169),first,last)
      | end
  MaxHwConf3 : Outport
  SelnCaseSt3 : Outport  Port=2
  wires:
  MaxHwConf2/1 -> MaxHwConf3/1
  SelnCaseSt2/1 -> SelnCaseSt3/1

== system SF042A_HwAgSnsrls/HwAgSnsrls/HwAgSnsrlsPer1/Arbitrator/MaxHwConf/If Action Subsystem4 ==
  StordHwConf : Inport
  Action Port : ActionPort  ActionType=else
  Constant2 : Constant  Value=LASTPOSNCON_CNT_U08
  CopyRight2 : Subsystem  Description=|  mask(Copyright Information){none=on}
      | Copyright info block.                                               
      |                                                                     
      | Place copyright information at the top of every subsystem in design.
      mask prompts: none "No parameters"
      mask help: Place copyright information at the top of every subsystem in design.
      mask Display:
      | NxtrConf = 'Nexteer Confidential';
      | 
      | sys = bdroot; %handle for the current model ("system")
      | first = get_param(sys,'Created');
      | if(isempty(first))
      |     first = datestr(now,'yyyy');
      | else
      |     first = first(end-3:end);  %year is last four digits
      | end
      | 
      | last = get_param(sys,'LastModifiedDate');
      | if isempty(last)
      |     last = datestr(now,'yyyy');
      | else
      |     last = last(end-3:end);
      | end
      | 
      | if strcmp(first,last)
      |     fprintf('%s -- Copyright %s Nexteer',NxtrConf,first)
      | else
      |     fprintf('%s -- %s%s- %s Nexteer',NxtrConf,char(169),first,last)
      | end
  MaxHwConf2 : Outport
  SelnCaseSt2 : Outport  Port=2
  wires:
  Constant2/1 -> SelnCaseSt2/1
  StordHwConf/1 -> MaxHwConf2/1
